simulink model "nid_spb_cvst_kinect_sdk_what_is_nid"  (Simulink 7.6)
settings: Solver=FixedStepDiscrete  StartTime=0.0  StopTime=inf  RelTol=1e-3
libraries: vipsnks x4, nid_lib x4, dspsrcs4 x1
settings Model: Creator=tchikama  LastModifiedBy=tchikama
settings DataIOCC: SaveOutput=off
settings OptimizationCC: SimCompilerOptimization=On
settings HardwareCC: ProdIntDivRoundTo=Zero  ProdEndianess=LittleEndian  ProdHWDeviceType=Generic->32-bit x86 compatible
settings RTWCC: ProcessScript=grt_make_rtw_hook  RTWCompilerOptimization=On
settings CodeAppCC: MaxIdLength=95

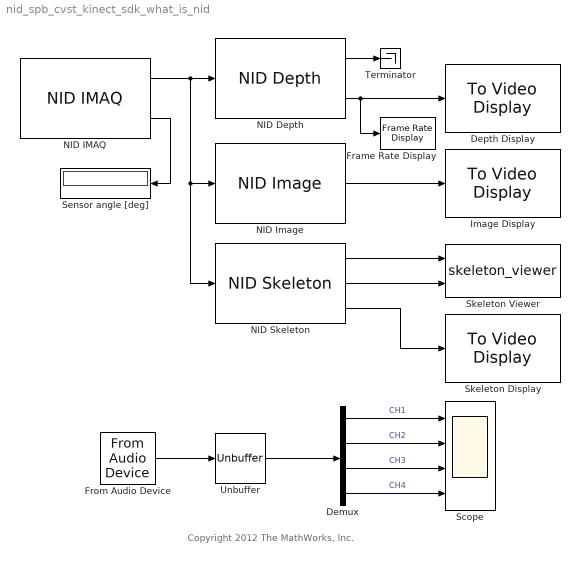
== system nid_spb_cvst_kinect_sdk_what_is_nid ==
  note: Copyright 2012 The MathWorks, Inc.
  Demux : Demux
  Depth Display : vipsnks/To Video Display  DialogControllerArgs=DataTag0  inputType=Obsolete  imagePorts=One multidimensional signal  OutputDevice=On-screen video monitor  fullScreen=off  videoWindowX=1124  videoWindowY=369  saveWindowSize=on  videoWindowWidth=377  videoWindowHeight=292  dataOrg=Column-major  openAtMdlStart=on  isWindowOpen=on
  Frame Rate Display : vipsnks/Frame Rate Display  DialogController=vipDDGCreate  DialogControllerArgs=DataTag1  UpdateRate=10
  From Audio Device : dspsrcs4/From Audio Device  DialogController=dspDDGCreate  DialogControllerArgs=DataTag2  deviceName=マイク配列 (Kinect USB Audio)  numChannels=4  sampleRate=16000  deviceDatatype=16-bit integer  autoBufferSize=on  bufferSize=4096  queueDuration=1.0  frameSize=1024  outputDatatype=single
  Image Display : vipsnks/To Video Display  DialogControllerArgs=DataTag3  inputType=Obsolete  imagePorts=One multidimensional signal  OutputDevice=On-screen video monitor  fullScreen=off  videoWindowX=1124  videoWindowY=24  saveWindowSize=on  videoWindowWidth=377  videoWindowHeight=292  dataOrg=Column-major  openAtMdlStart=on  isWindowOpen=on
  NID Depth : nid_lib/NID Depth  depthOutput=Depth  conv_XYZ_RW=off  viewer=on
  NID IMAQ : nid_lib/NID IMAQ  imaq_depth=on  imaq_motion=off  imaq_image=on  view_point=on  imaq_skeleton=on  imaq_ir=off  mirror_image=off  imaq_sample_time=1/30  res_fps=VGA (640x480): 30 FPS  needPsiPose=off  angle=0  angle_read=on  near_mode=off
  NID Image : nid_lib/NID Image  imageOutput=RGB
  NID Skeleton : nid_lib/NID Skeleton  num_of_skeleton_tracking=1  conv_XYZ_RW=on  viewer=on
  Scope : Scope  NumInputPorts=4
      settings: TimeRange=10  YMin=-2~-2~-2~-2  YMax=2~2~2~2
  Sensor angle [deg] : Display
  Skeleton Display : vipsnks/To Video Display  DialogControllerArgs=DataTag4  inputType=Obsolete  imagePorts=One multidimensional signal  OutputDevice=On-screen video monitor  fullScreen=off  videoWindowX=172  videoWindowY=25  saveWindowSize=on  videoWindowWidth=377  videoWindowHeight=292  dataOrg=Column-major  openAtMdlStart=on  isWindowOpen=on
  Skeleton Viewer : M-S-Function  FunctionName=skeleton_viewer
      mask Display:
      | disp('Skeleton\nViewer')
      | 
      | port_label('input', 1, 'Tracking')
      | port_label('input', 2, 'Skeleton')
  Terminator : Terminator
  Unbuffer : Unbuffer  SampleBasedProcessing=Same as frame based
  wires:
  NID IMAQ/1 -> NID Depth/1, NID Skeleton/1, NID Image/1
  NID Skeleton/1 -> Skeleton Viewer/1
  NID Skeleton/2 -> Skeleton Viewer/2
  NID Skeleton/3 -> Skeleton Display/1
  NID Depth/2 -> Depth Display/1, Frame Rate Display/1
  NID Depth/1 -> Terminator/1
  NID Image/1 -> Image Display/1
  From Audio Device/1 -> Unbuffer/1
  Unbuffer/1 -> Demux/1
  Demux/1 -> Scope/1  "CH1"
  Demux/2 -> Scope/2  "CH2"
  Demux/3 -> Scope/3  "CH3"
  Demux/4 -> Scope/4  "CH4"
  NID IMAQ/2 -> Sensor angle [deg]/1
